simulink model "ModelVls"  (R2022b)
settings: Solver=FixedStepDiscrete  StartTime=0.0  StopTime=1  RelTol=1e-3  EnableMultiTasking=on
InitFcn:
  | % Initialize model
  | run([ModelRootName() 'Init.m']);
  | 
  | % load library data
  | GainLibrary_data;
StartFcn:
  | % make sure all the simulated RTC requests are found
  | %RTC_SIM_OBJ.ValidateREQs();
model workspace (MAT data in the model file):
  PreampVolumeTable_Idx : Simulink.Signal (value not decoded)
  Range : Simulink.Signal (value not decoded)
  Table_Idx : Simulink.Signal (value not decoded)
undefined symbols (not defined in the file): Config, Ifir, IFIR, MedusaConfig, MuteRamper, MuteRamperBtc, numAudioIn, preAmp, Row, sys_defs, VLSConfig
libraries: FeaturePath x22, TuneVar x17, RTC x9, MedusaDelays x9, dspindex x5, TOP x5, SampleRateConverter x4, EdgePorts x2, PooliirLib x2, MedusaCaeEnable x2, FIREven x2, VLSGains x2
(part 2 of 4)

== system ModelVls/PreAmp/DecRate/Medusa5H1/MedusaHoligram/Medusa5H1 Part 2 ==
  AudioIn : Inport  OutDataTypeStr=single
  LRbp : Inport  Port=2
  LRhp : Inport  Port=3
  CAEEnable : Inport  Port=4
  Alignment Delay : Subsystem  TreatAsAtomicUnit=on
      settings: RTWSystemCode=Nonreusable function  FunctionWithSeparateData=on
  Decimated-Rate FDP : MedusaFDP/Decimated-Rate  FeatureName=DeciRate  configStruct=config.DRFDPConfig  RfftConfig=[]  RifftConfig=[]
  Full-Rate FDP : MedusaFullRateFDP/Full-Rate  FeatureName=FullRate  configStruct=config.FRFDPConfig  RfftConfig=[]  RifftConfig=[]
  Mono Detector : MonoDetector/MedusaMonoDetector  Config=Config.MonoDetector
  Partition : FeaturePath/Partition  PartitionNumber=3  TriggerInit=[825 236 870 304]
      settings: SourceProductName=Bose Talaria
  SPUM Decay Estimate : MedusaSPUMDecayEst/SPUM Decay Estimate  configStruct=config.FRFDPConfig
  Selector : Selector  NumberOfDimensions=2  InputPortWidth=3  IndexOptions=Select all,Index vector (dialog)  Indices=[1 3],[1,2]  OutputSizes=1,1
  Selector1 : Selector  NumberOfDimensions=2  InputPortWidth=3  IndexOptions=Select all,Index vector (dialog)  Indices=[1 3],[1 2 3 5]  OutputSizes=1,1
  DRComps : Outport  VectorParamsAs1DForOutWhenUnconnected=off
  FRComps : Outport  Port=2  VectorParamsAs1DForOutWhenUnconnected=off
  HFRef : Outport  Port=3
  wires:
  Alignment Delay/1(LRtreble) -> Full-Rate FDP/1
  CAEEnable/1 -> Full-Rate FDP/2, Decimated-Rate FDP/2
  Selector1/1 -> HFRef/1  "Lo, Ro, Limp, Rimp"
  Full-Rate FDP/1 -> FRComps/1, Selector1/1  "Lo, Ro, Limp, Ltail, Rimp, Rtail"
  [isStereo] -> SPUM Decay Estimate/2
  LRhp/1 -> SPUM Decay Estimate/1, Alignment Delay/1(LRhp)
  LRbp/1 -> Decimated-Rate FDP/1
  AudioIn/1 -> Selector/1
  Selector/1 -> Mono Detector/1  "L, R"
  Mono Detector/1 -> [isStereo]
  SPUM Decay Estimate/1 -> Decimated-Rate FDP/3, Full-Rate FDP/3
  Decimated-Rate FDP/1 -> DRComps/1  "Lo, Ro, Ls, Rs, Limp, Ltail, Rimp, Rtail"

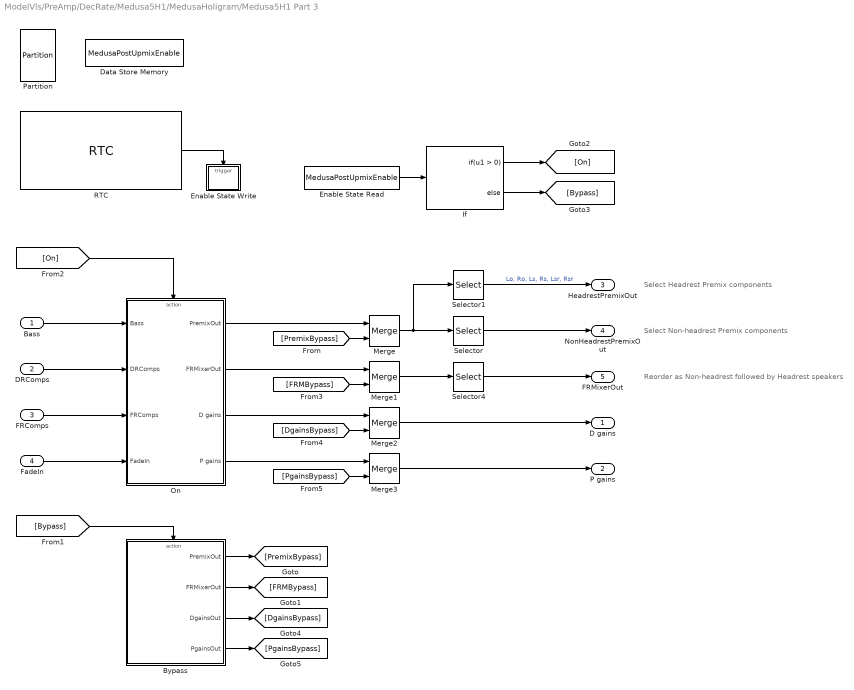
== system ModelVls/PreAmp/DecRate/Medusa5H1/MedusaHoligram/Medusa5H1 Part 3 ==
  note: Select Headrest Premix components
  note: Select Non-headrest Premix components
  note: Reorder as Non-headrest followed by Headrest speakers
  Bass : Inport
  DRComps : Inport  Port=2
  FRComps : Inport  Port=3
  FadeIn : Inport  Port=4
  Bypass : Subsystem
  Data Store Memory : DataStoreMemory  DataStoreName=MedusaPostUpmixEnable  ReadBeforeWriteMsg=warning  WriteAfterWriteMsg=warning  WriteAfterReadMsg=warning  InitialValue=1  ShowAdditionalParam=off  OutDataTypeStr=uint32
  Enable State Read : DataStoreRead  DataStoreName=MedusaPostUpmixEnable  IndexOptions=Index vector (dialog)  Indices=1  OutputSizes=1
  Enable State Write : Subsystem
  If : If
  Merge : Merge  InitialOutput=zeros(config.HoligramEQConfig.frameSize, config.PremixConfig.NumPremixOut)
  Merge1 : Merge  InitialOutput=Config.DefaultFullRateMixerOutput
  Merge2 : Merge  InitialOutput=zeros(config.numVLSGains, 1)
  Merge3 : Merge  InitialOutput=zeros(config.numVLSGains, 1)
  On : Subsystem
  Partition : FeaturePath/Partition  PartitionNumber=5  TriggerInit=[410 331 455 399]
      settings: SourceProductName=Bose Talaria
  RTC : RTC/RTC  REQ_Priority=RTC_Mask.NormalPriority  RequestAtInit=off  EnableRequest=on  REQElemType1=int32  REQElemWidth1=1  REQElemInitial1=[]  REQElemType2=uint32  REQElemWidth2=1  REQElemInitial2=[]  REQElemType3=uint32  REQElemWidth3=1  REQElemInitial3=[]  REQElemType4=uint32  REQElemWidth4=1  REQElemInitial4=[]  REQElemType5=uint32  REQElemWidth5=1  REQElemInitial5=[]  REQElemType6=uint32  REQElemWidth6=1  REQElemInitial6=[]  REQElemType7=uint32  REQElemWidth7=1  REQElemInitial7=[]  REQElemType8=uint32  REQElemWidth8=1  REQElemInitial8=[]  REQElemType9=uint32  REQElemWidth9=1  REQElemInitial9=[]  REQElemType10=uint32  REQElemWidth10=1  REQElemInitial10=[]  EnableResponse=on  EnableRSP_StatusIn=off  RSPElemType1=uint32  RSPElemWidth1=1  RSPElemType2=uint32  RSPElemWidth2=1  RSPElemType3=uint32  RSPElemWidth3=1  RSPElemType4=uint32  RSPElemWidth4=1  RSPElemType5=uint32  RSPElemWidth5=1  RSPElemType6=uint32  RSPElemWidth6=1  RSPElemType7=uint32  RSPElemWidth7=1  RSPElemType8=uint32  RSPElemWidth8=1  RSPElemType9=uint32  RSPElemWidth9=1  RSPElemType10=uint32  RSPElemWidth10=1  EnableNotification=off  EnableNTF_PrepTrig=off  NTFElemType1=uint32  NTFElemWidth1=1  NTFElemType2=uint32  NTFElemWidth2=1  NTFElemType3=uint32  NTFElemWidth3=1  NTFElemType4=uint32  NTFElemWidth4=1  NTFElemType5=uint32  NTFElemWidth5=1  NTFElemType6=uint32  NTFElemWidth6=1  NTFElemType7=uint32  NTFElemWidth7=1  NTFElemType8=uint32  NTFElemWidth8=1  NTFElemType9=uint32  NTFElemWidth9=1  NTFElemType10=uint32  NTFElemWidth10=1  MaskMessageName=PostUpmixDisable
      settings: SourceProductName=Bose Talaria
  Selector : Selector  NumberOfDimensions=2  InputPortWidth=3  IndexOptions=Select all,Index vector (dialog)  Indices=[1 3],config.NonHeadrestIdx  OutputSizes=1,1
  Selector1 : Selector  NumberOfDimensions=2  InputPortWidth=3  IndexOptions=Select all,Index vector (dialog)  Indices=[1 3],config.HeadrestIdx  OutputSizes=1,1
  Selector4 : Selector  NumberOfDimensions=2  InputPortWidth=3  IndexOptions=Select all,Index vector (dialog)  Indices=[1 3],config.FRMOutputIdx  OutputSizes=1,1
  D gains : Outport
  P gains : Outport  Port=2
  HeadrestPremixOut : Outport  Port=3  VectorParamsAs1DForOutWhenUnconnected=off
  NonHeadrestPremixOut : Outport  Port=4  VectorParamsAs1DForOutWhenUnconnected=off
  FRMixerOut : Outport  Port=5  VectorParamsAs1DForOutWhenUnconnected=off
  wires:
  Selector1/1 -> HeadrestPremixOut/1  "Lo, Ro, Ls, Rs, Lsr, Rsr"
  Selector/1 -> NonHeadrestPremixOut/1
  Merge3/1 -> P gains/1
  Merge2/1 -> D gains/1
  On/4(P gains) -> Merge3/1
  On/3(D gains) -> Merge2/1
  Merge1/1 -> Selector4/1
  On/2(FRMixerOut) -> Merge1/1
  RTC/1 -> Enable State Write/Trigger
  [On] -> On/Action
  Enable State Read/1 -> If/1
  If/2 -> [Bypass]
  If/1 -> [On]
  Merge/1 -> Selector/1, Selector1/1
  On/1(PremixOut) -> Merge/1
  [Bypass] -> Bypass/Action
  DRComps/1 -> On/2(DRComps)
  Bass/1 -> On/1(Bass)
  FRComps/1 -> On/3(FRComps)
  FadeIn/1 -> On/4(FadeIn)
  Bypass/1(PremixOut) -> [PremixBypass]
  Bypass/2(FRMixerOut) -> [FRMBypass]
  Bypass/3(DgainsOut) -> [DgainsBypass]
  Bypass/4(PgainsOut) -> [PgainsBypass]
  [PremixBypass] -> Merge/2
  [FRMBypass] -> Merge1/2
  [DgainsBypass] -> Merge2/2
  [PgainsBypass] -> Merge3/2
  Selector4/1 -> FRMixerOut/1

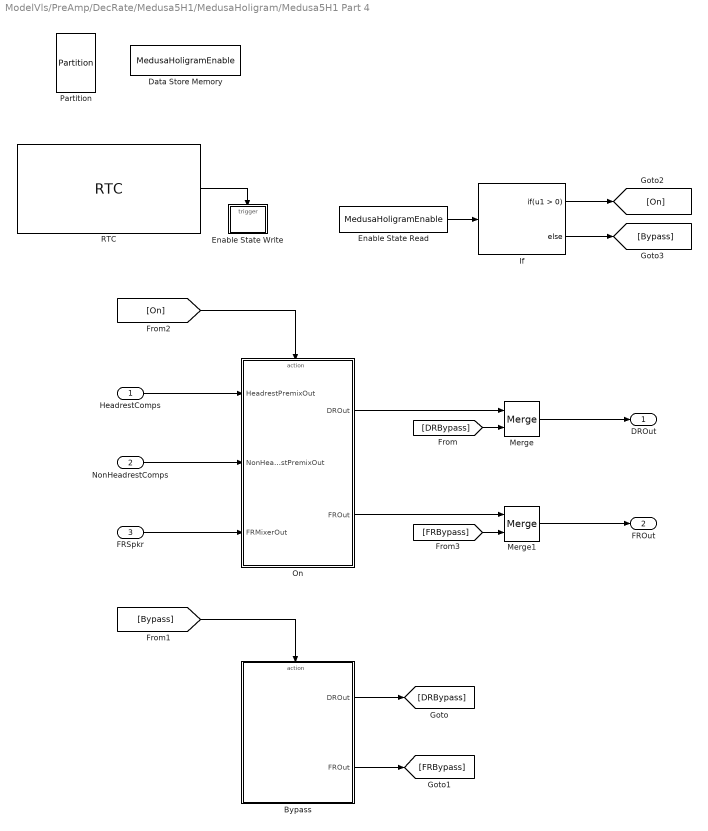
== system ModelVls/PreAmp/DecRate/Medusa5H1/MedusaHoligram/Medusa5H1 Part 4 ==
  HeadrestComps : Inport
  NonHeadrestComps : Inport  Port=2
  FRSpkr : Inport  Port=3
  Bypass : Subsystem
  Data Store Memory : DataStoreMemory  DataStoreName=MedusaHoligramEnable  ReadBeforeWriteMsg=warning  WriteAfterWriteMsg=warning  WriteAfterReadMsg=warning  InitialValue=1  ShowAdditionalParam=off  OutDataTypeStr=uint32
  Enable State Read : DataStoreRead  DataStoreName=MedusaHoligramEnable  IndexOptions=Index vector (dialog)  Indices=1  OutputSizes=1
  Enable State Write : Subsystem
  If : If
  Merge : Merge  InitialOutput=zeros(config.HoligramEQConfig.frameSize, config.numDRChan)
  Merge1 : Merge  InitialOutput=zeros(config.HoligramEQConfig.frameSizeFR, config.numMedusaOut)
  On : Subsystem
  Partition : FeaturePath/Partition  PartitionNumber=6  TriggerInit=[335 311 380 379]
      settings: SourceProductName=Bose Talaria
  RTC : RTC/RTC  REQ_Priority=RTC_Mask.NormalPriority  RequestAtInit=off  EnableRequest=on  REQElemType1=int32  REQElemWidth1=1  REQElemInitial1=[]  REQElemType2=uint32  REQElemWidth2=1  REQElemInitial2=[]  REQElemType3=uint32  REQElemWidth3=1  REQElemInitial3=[]  REQElemType4=uint32  REQElemWidth4=1  REQElemInitial4=[]  REQElemType5=uint32  REQElemWidth5=1  REQElemInitial5=[]  REQElemType6=uint32  REQElemWidth6=1  REQElemInitial6=[]  REQElemType7=uint32  REQElemWidth7=1  REQElemInitial7=[]  REQElemType8=uint32  REQElemWidth8=1  REQElemInitial8=[]  REQElemType9=uint32  REQElemWidth9=1  REQElemInitial9=[]  REQElemType10=uint32  REQElemWidth10=1  REQElemInitial10=[]  EnableResponse=on  EnableRSP_StatusIn=off  RSPElemType1=uint32  RSPElemWidth1=1  RSPElemType2=uint32  RSPElemWidth2=1  RSPElemType3=uint32  RSPElemWidth3=1  RSPElemType4=uint32  RSPElemWidth4=1  RSPElemType5=uint32  RSPElemWidth5=1  RSPElemType6=uint32  RSPElemWidth6=1  RSPElemType7=uint32  RSPElemWidth7=1  RSPElemType8=uint32  RSPElemWidth8=1  RSPElemType9=uint32  RSPElemWidth9=1  RSPElemType10=uint32  RSPElemWidth10=1  EnableNotification=off  EnableNTF_PrepTrig=off  NTFElemType1=uint32  NTFElemWidth1=1  NTFElemType2=uint32  NTFElemWidth2=1  NTFElemType3=uint32  NTFElemWidth3=1  NTFElemType4=uint32  NTFElemWidth4=1  NTFElemType5=uint32  NTFElemWidth5=1  NTFElemType6=uint32  NTFElemWidth6=1  NTFElemType7=uint32  NTFElemWidth7=1  NTFElemType8=uint32  NTFElemWidth8=1  NTFElemType9=uint32  NTFElemWidth9=1  NTFElemType10=uint32  NTFElemWidth10=1  MaskMessageName=HoligramDisable
      settings: SourceProductName=Bose Talaria
  DROut : Outport  VectorParamsAs1DForOutWhenUnconnected=off
  FROut : Outport  Port=2  VectorParamsAs1DForOutWhenUnconnected=off
  wires:
  Merge1/1 -> FROut/1
  On/2(FROut) -> Merge1/1
  RTC/1 -> Enable State Write/Trigger
  [On] -> On/Action
  Enable State Read/1 -> If/1
  If/2 -> [Bypass]
  If/1 -> [On]
  Merge/1 -> DROut/1
  On/1(DROut) -> Merge/1
  [Bypass] -> Bypass/Action
  FRSpkr/1 -> On/3(FRMixerOut)
  NonHeadrestComps/1 -> On/2(NonHeadrestPremixOut)
  HeadrestComps/1 -> On/1(HeadrestPremixOut)
  Bypass/1(DROut) -> [DRBypass]
  Bypass/2(FROut) -> [FRBypass]
  [DRBypass] -> Merge/2
  [FRBypass] -> Merge1/2

== system ModelVls/PreAmp/DecRate/Medusa5H1/MedusaHoligram/Medusa5H1 Part 5 ==
  DRIn : Inport
  FRIn : Inport  Port=2
  DR Speaker and HRComps Delay : MedusaDelays/MedusaTunableDelay  Config=Config.DeciRateSpeakerDelay
  FR Speaker Delay : MedusaDelays/MedusaTunableDelay  Config=Config.FullRateSpeakerDelay
  Partition : FeaturePath/Partition  PartitionNumber=7  TriggerInit=[1360 586 1405 654]
      settings: SourceProductName=Bose Talaria
  Speaker Delay Tune : Subsystem
  DROut : Outport  VectorParamsAs1DForOutWhenUnconnected=off
  FROut : Outport  Port=2  VectorParamsAs1DForOutWhenUnconnected=off
  wires:
  DR Speaker and HRComps Delay/1 -> DROut/1
  Speaker Delay Tune/2(FRSpeakerDelay) -> [FRSpeakerDelay]
  [DRSpeakerDelay] -> DR Speaker and HRComps Delay/2
  Speaker Delay Tune/1(DRSpeakerDelay) -> [DRSpeakerDelay]
  [FRSpeakerDelay] -> FR Speaker Delay/2
  FR Speaker Delay/1 -> FROut/1
  FRIn/1 -> FR Speaker Delay/1
  DRIn/1 -> DR Speaker and HRComps Delay/1

== system ModelVls/PreAmp/DecRate/Medusa5H1/PreAmpPart2/MuteRamperDR ==
  AudioIn : Inport
  REQ : Inport  Port=2
  NTF : Inport  Port=3
  Bus Element In2 : Inport  Port=4
  InnerLink : Subsystem  AncestorBlock=MuteRamperBtc/MuteRamper  mask(Blocklib MuteRamper){Config=InnerLinkConfig}
      mask prompts: Config "MuteRamperConfig"
      mask help: This component is to be used in conjunction with the MuteControl block, which provides runtime control and tuning capabilities via an RTC and the tune variable muteControlRampTime. Multiple instances of this block may be placed within an audio application, and a single MuteControl block has the ability to control all of these rampers simultaneously.
      mask init:
      | blkh=gcbh;
      | Config=BTConfig.Assert(blkh,Config);
      | Config.Validate();
      | 
      | % Set boundary conditions
      | rampRateBounds = [5,50000];
      | rampTimeBounds = [1,3000];
      | 
      | % Setup Dsms
      | theDsms = {'currentGain','targetLinearGain','nFrames'};
      | CscUtil.SetupDsmsForStaticInit(blkh,theDsms);
      settings: LibrarySourceBlock=MuteRamperBtc/MuteRamper
  audioOut : Outport
  NTF_check : Outport  Port=2
  wires:
  Bus Element In2/1 -> InnerLink/4(InBus)
  NTF/1 -> InnerLink/3(NTF)
  REQ/1 -> InnerLink/2(REQ)
  AudioIn/1 -> InnerLink/1(AudioIn)
  InnerLink/2(NTF_check) -> NTF_check/1
  InnerLink/1(audioOut) -> audioOut/1

== system ModelVls/PreAmp/DecRate/Medusa5H1/PreAmpPart2/MuteRamperFR ==
  AudioIn : Inport
  REQ : Inport  Port=2
  NTF : Inport  Port=3
  Bus Element In2 : Inport  Port=4
  InnerLink : Subsystem  AncestorBlock=MuteRamperBtc/MuteRamper  mask(Blocklib MuteRamper){Config=InnerLinkConfig}
      mask prompts: Config "MuteRamperConfig"
      mask help: This component is to be used in conjunction with the MuteControl block, which provides runtime control and tuning capabilities via an RTC and the tune variable muteControlRampTime. Multiple instances of this block may be placed within an audio application, and a single MuteControl block has the ability to control all of these rampers simultaneously.
      mask init: same as ModelVls/PreAmp/DecRate/Medusa5H1/PreAmpPart2/MuteRamperDR/InnerLink
      settings: LibrarySourceBlock=MuteRamperBtc/MuteRamper
  audioOut : Outport
  NTF_check : Outport  Port=2
  wires:
  Bus Element In2/1 -> InnerLink/4(InBus)
  NTF/1 -> InnerLink/3(NTF)
  REQ/1 -> InnerLink/2(REQ)
  AudioIn/1 -> InnerLink/1(AudioIn)
  InnerLink/2(NTF_check) -> NTF_check/1
  InnerLink/1(audioOut) -> audioOut/1

== system ModelVls/PreAmp/DecRate/Medusa5H1/PreAmpPart2/Subsystem ==
  In1 : Inport
  Inport : Inport  Port=2
  Trigger : TriggerPort  TriggerType=function-call  VariantControl=Variant  PortDimensions=1
  AND : Logic  IconShape=distinctive  AllPortsSameDT=off  OutDataTypeStr=boolean
  Out1 : Outport
  wires:
  In1/1 -> AND/1
  AND/1 -> Out1/1
  Inport/1 -> AND/2

== system ModelVls/PreAmp/DecRate/Medusa5H1/PreAmpPart2/Subsystem1 ==
  In1 : Inport
  Inport : Inport  Port=2
  Trigger : TriggerPort  TriggerType=function-call  VariantControl=Variant  PortDimensions=1
  AND : Logic  IconShape=distinctive  AllPortsSameDT=off  OutDataTypeStr=boolean
  Out1 : Outport
  wires:
  In1/1 -> AND/1
  AND/1 -> Out1/1
  Inport/1 -> AND/2

== system ModelVls/PreAmp/DecRate/Medusa5H1/MedusaHoligram/Medusa5H1 Part 1/CAE Treble Boost ==
  note: 1) Add Subsystem or Model blocks as valid variant choices.
      | 2) You cannot connect blocks at this level. At simulation, connectivity is automatically
      | determined, based on the active variant and port name matching.
  AudioIn : Inport
  Audio Passthrough : Subsystem  VariantControl=sys_defs.include_compressed_audio_enhancement == 0
  "CAE Treble Boost " : Subsystem  VariantControl=sys_defs.include_compressed_audio_enhancement == 1
  Out : Outport
  CAEEnable : Outport  Port=2

== system ModelVls/PreAmp/DecRate/Medusa5H1/MedusaHoligram/Medusa5H1 Part 1/Medusa Band Split Stereo ==
  LRhp : Inport
  Band Separation Delay : Delay  DelayLength=configStruct.band_separation_delay  InputProcessing=Columns as channels (frame based)
  Constant : Constant  Value=zeros(numInputs, 1)  OutDataTypeStr=uint32
  Downsample : DownSample  N=configStruct.D
  Image Rejection Filter : FIREven/FIR Even  variantSelect=Hexagon
      settings: SourceProductName=Bose Blocklib
  Image Rejection Filter Coeffs : Constant  Value=configStruct.fireven
  Interpolated Filter : Subsystem  AncestorBlock=Ifir/IFIR  mask(Interpolated FIR){coeffsFlip=configStruct.ifir, I=configStruct.D/2, numChannels=numInputs}
      mask prompts: coeffsFlip "Coefficients"; I "Interpolation Factor"; numChannels "Num inputs"
      mask help:
      | An interpolated FIR filter is an FIR filter with a sparse set of coefficients containing I-1 zeros between each point, where I is the interpolation factor.
      |
      | The block supports multiple channels, with each channel sharing the same set of filter coefficients. Users need to specify the non-zero coefficients, the interpolation factor and the number of channels.
      mask init:
      | % Flip the coeffs
      | [~, numCoeffSets] = size(coeffsFlip);
      | ind = 0:numCoeffSets-1;
      | coeffsFlip = flipud(coeffsFlip(:,ind+1));
      | 
      | % Cast decimation factor to int32
      | I = int32(I);
      settings: LibrarySourceBlock=Ifir/IFIR
  Reconstruction Filter : dspmlti4/FIR Interpolation  FilterSource=Dialog parameters  PrivateCoeffs=0  h=configStruct.upfir  L=configStruct.D  FilterObject=FINTERP  InputProcessing=Columns as channels (frame based)  framing=Enforce single-rate processing  outputBufInitCond=0  roundingMode=Floor  overflowMode=off  firstCoeffDataTypeStr=Inherit: Same word length as input  firstCoeffMin=[]  firstCoeffMax=[]  firstCoeffLastDataTypeStr=Inherit: Same word length as input  outputDataTypeStr=Inherit: Same as accumulator  outputMin=[]  outputMax=[]  outputLastDataTypeStr=Inherit: Same as accumulator
  Sum : Sum  Inputs=-+|
  LRbp : Outport  VectorParamsAs1DForOutWhenUnconnected=off
  LRtreble : Outport  Port=2  VectorParamsAs1DForOutWhenUnconnected=off
  wires:
  Constant/1 -> Image Rejection Filter/3
  Reconstruction Filter/1 -> Sum/1
  Interpolated Filter/1(AudioOut) -> Image Rejection Filter/1
  LRhp/1 -> Interpolated Filter/1(AudioIn), Band Separation Delay/1
  Image Rejection Filter Coeffs/1 -> Image Rejection Filter/2
  Image Rejection Filter/1 -> Downsample/1
  Sum/1 -> LRtreble/1
  Band Separation Delay/1 -> Sum/2
  Downsample/1 -> Reconstruction Filter/1, LRbp/1

== system ModelVls/PreAmp/DecRate/Medusa5H1/MedusaHoligram/Medusa5H1 Part 2/Alignment Delay ==
  LRhp : Inport
  Full-rate Alignment Delay Translation : MedusaDelays/MedusaFullRateAlignmentDelayTranslation  Config=Config.TrebleDelayTranslation
  Treble Delay : MedusaDelays/MedusaAlignmentDelay  Config=Config.TrebleDelay
  Tune Variable1 : TuneVar/TuneVar  TuneName=DeciRateNearWiggleFilterDelaySamples  SpecifyMaxSize=off  VariableDim=1 (Row)  MaxSize=[1 1]  TunabilityNumber=1  MinValue=[]  MaxValue=[]  TriggerInit=[-15 450 150 500]  MaskValue=Config.TrebleDelayTranslation.DefaultTuning.DeciRateNearWiggleDelay
      settings: SourceProductName=Bose Talaria
  Tune Variable4 : TuneVar/TuneVar  TuneName=DeciRateWiggleFilterDelaySamples  SpecifyMaxSize=off  VariableDim=1 (Row)  MaxSize=[1 1]  TunabilityNumber=1  MinValue=[]  MaxValue=[]  TriggerInit=[-15 385 150 435]  MaskValue=Config.TrebleDelayTranslation.DefaultTuning.DeciRateWiggleDelay
      settings: SourceProductName=Bose Talaria
  Tune Variable5 : TuneVar/TuneVar  TuneName=HoligramFilterAlignmentDelaySamples  SpecifyMaxSize=off  VariableDim=1 (Row)  MaxSize=[1 1]  TunabilityNumber=1  MinValue=[]  MaxValue=[]  TriggerInit=[-15 515 150 565]  MaskValue=Config.TrebleDelayTranslation.DefaultTuning.HoligramDelay
      settings: SourceProductName=Bose Talaria
  LRtreble : Outport
  wires:
  Tune Variable1/1 -> Full-rate Alignment Delay Translation/2  "DeciRateNearWiggleFilterDelaySamples"
  Tune Variable5/1 -> Full-rate Alignment Delay Translation/3  "HoligramFilterAlignmentDelaySamples"
  LRhp/1 -> Treble Delay/1
  Tune Variable4/1 -> Full-rate Alignment Delay Translation/1  "DeciRateWiggleFilterDelaySamples"
  Full-rate Alignment Delay Translation/1 -> [TrebleDelay]
  [TrebleDelay] -> Treble Delay/2
  Treble Delay/1 -> LRtreble/1  "LRtreble"

== system ModelVls/PreAmp/DecRate/Medusa5H1/MedusaHoligram/Medusa5H1 Part 3/Bypass ==
  Action Port : ActionPort  ActionPortLabel=else
  Constant : Constant  Value=zeros(config.HoligramEQConfig.frameSize, config.PremixConfig.NumPremixOut)  OutDataTypeStr=single
  Constant1 : Constant  Value=Config.DefaultFullRateMixerOutput  OutDataTypeStr=single
  Constant2 : Constant  Value=zeros(config.numVLSGains, 1)  OutDataTypeStr=single
  Constant3 : Constant  Value=zeros(config.numVLSGains, 1)  OutDataTypeStr=single
  PremixOut : Outport  VectorParamsAs1DForOutWhenUnconnected=off
  FRMixerOut : Outport  Port=2  VectorParamsAs1DForOutWhenUnconnected=off
  DgainsOut : Outport  Port=3  VectorParamsAs1DForOutWhenUnconnected=off
  PgainsOut : Outport  Port=4  VectorParamsAs1DForOutWhenUnconnected=off
  wires:
  Constant2/1 -> DgainsOut/1
  Constant3/1 -> PgainsOut/1
  Constant1/1 -> FRMixerOut/1
  Constant/1 -> PremixOut/1

== system ModelVls/PreAmp/DecRate/Medusa5H1/MedusaHoligram/Medusa5H1 Part 3/Enable State Write ==
  Trigger : TriggerPort  TriggerType=function-call  VariantControl=Variant  PortDimensions=1
  Constant : Constant  Value=0  OutDataTypeStr=uint32
  Data Store Write : DataStoreWrite  DataStoreName=MedusaPostUpmixEnable  IndexOptions=Index vector (dialog)  Indices=1  OutputSizes=1
  wires:
  Constant/1 -> Data Store Write/1

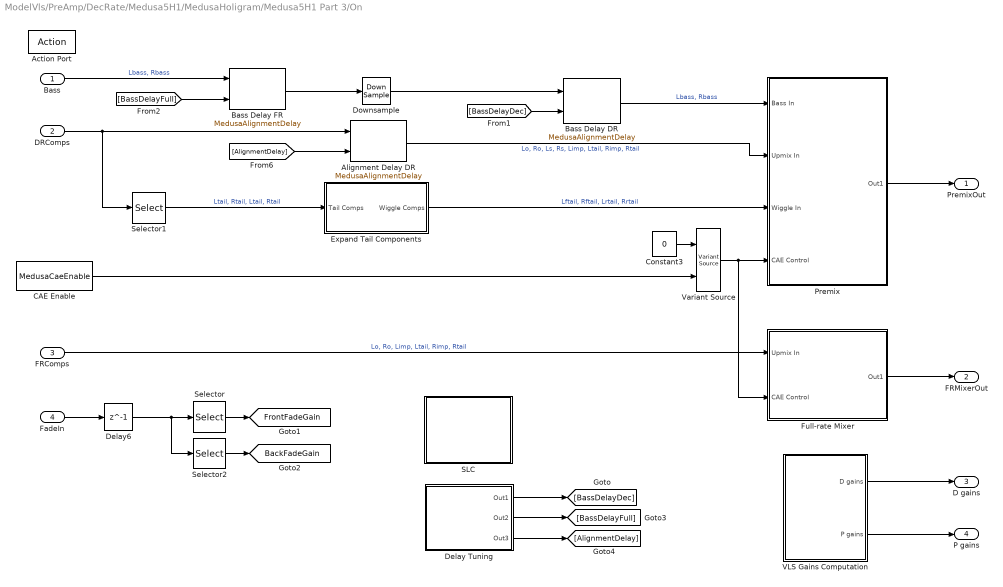
== system ModelVls/PreAmp/DecRate/Medusa5H1/MedusaHoligram/Medusa5H1 Part 3/On ==
  Bass : Inport  OutDataTypeStr=single
  DRComps : Inport  Port=2  OutDataTypeStr=single
  FRComps : Inport  Port=3  OutDataTypeStr=single
  FadeIn : Inport  Port=4  OutDataTypeStr=single
  Action Port : ActionPort  ActionPortLabel=if(u1 > 0)
  Alignment Delay DR : MedusaDelays/MedusaAlignmentDelay  Config=Config.MidrangeDelay
  Bass Delay DR : MedusaDelays/MedusaAlignmentDelay  Config=Config.DeciRateBassDelay
  Bass Delay FR : MedusaDelays/MedusaAlignmentDelay  Config=Config.FullRateBassDelay
  CAE Enable : MedusaCaeEnable/MedusaCaeEnable  Config=Config.PremixCaeEnable  MaskMessageName=PremixCAEEnable
  Constant3 : Constant  Value=0  OutDataTypeStr=int32  SampleTime=-1
  Delay Tuning : Subsystem
  Delay6 : Delay  DelayLength=1
  Downsample : DownSample  N=4
  Expand Tail Components : Subsystem  TreatAsAtomicUnit=on  RTWFileName=MedusaExpandTailComps
      settings: RTWSystemCode=Nonreusable function  RTWFileNameOpts=User specified  FunctionWithSeparateData=on
  Full-rate Mixer : Subsystem
  Premix : Subsystem
  SLC : Subsystem
  Selector : Selector  NumberOfDimensions=2  InputPortWidth=2  IndexOptions=Index vector (dialog),Index vector (dialog)  Indices=1,1  OutputSizes=1,1
  Selector1 : Selector  NumberOfDimensions=2  InputPortWidth=3  IndexOptions=Select all,Index vector (dialog)  Indices=[1 3],[6 8 6 8]  OutputSizes=1,1
  Selector2 : Selector  NumberOfDimensions=2  InputPortWidth=2  IndexOptions=Index vector (dialog),Index vector (dialog)  Indices=1,2  OutputSizes=1,1
  VLS Gains Computation : Subsystem
  Variant Source : VariantSource
  PremixOut : Outport  VectorParamsAs1DForOutWhenUnconnected=off
  FRMixerOut : Outport  Port=2  VectorParamsAs1DForOutWhenUnconnected=off
  D gains : Outport  Port=3
  P gains : Outport  Port=4
  tag scope: BackFadeGain=global, FrontFadeGain=global
  wires:
  Alignment Delay DR/1 -> Premix/2(Upmix In)  "Lo, Ro, Ls, Rs, Limp, Ltail, Rimp, Rtail"
  Variant Source/1 -> Full-rate Mixer/2(CAE Control), Premix/4(CAE Control)
  Constant3/1 -> Variant Source/1
  CAE Enable/1 -> Variant Source/2
  Full-rate Mixer/1(Out1) -> FRMixerOut/1
  FRComps/1 -> Full-rate Mixer/1(Upmix In)  "Lo, Ro, Limp, Ltail, Rimp, Rtail"
  Premix/1(Out1) -> PremixOut/1
  Expand Tail Components/1(Wiggle Comps) -> Premix/3(Wiggle In)  "Lftail, Rftail, Lrtail, Rrtail"
  Bass Delay DR/1 -> Premix/1(Bass In)  "Lbass, Rbass"
  VLS Gains Computation/2(P gains) -> P gains/1
  VLS Gains Computation/1(D gains) -> D gains/1
  Delay Tuning/3(Out3) -> [AlignmentDelay]
  Delay Tuning/2(Out2) -> [BassDelayFull]
  Delay Tuning/1(Out1) -> [BassDelayDec]
  DRComps/1 -> Alignment Delay DR/1, Selector1/1
  Downsample/1 -> Bass Delay DR/1
  [BassDelayDec] -> Bass Delay DR/2
  [AlignmentDelay] -> Alignment Delay DR/2
  [BassDelayFull] -> Bass Delay FR/2
  Bass/1 -> Bass Delay FR/1  "Lbass, Rbass"
  Selector1/1 -> Expand Tail Components/1(Tail Comps)  "Ltail, Rtail, Ltail, Rtail"
  Bass Delay FR/1 -> Downsample/1
  FadeIn/1 -> Delay6/1
  Selector2/1 -> [BackFadeGain]
  Delay6/1 -> Selector2/1, Selector/1
  Selector/1 -> [FrontFadeGain]

== system ModelVls/PreAmp/DecRate/Medusa5H1/MedusaHoligram/Medusa5H1 Part 4/Bypass ==
  Action Port : ActionPort  ActionPortLabel=else
  Constant : Constant  Value=zeros(config.HoligramEQConfig.frameSize, config.numDRChan)  OutDataTypeStr=single
  Constant1 : Constant  Value=zeros(config.HoligramEQConfig.frameSizeFR, config.numMedusaOut)  OutDataTypeStr=single
  DROut : Outport  VectorParamsAs1DForOutWhenUnconnected=off
  FROut : Outport  Port=2  VectorParamsAs1DForOutWhenUnconnected=off
  wires:
  Constant1/1 -> FROut/1
  Constant/1 -> DROut/1

== system ModelVls/PreAmp/DecRate/Medusa5H1/MedusaHoligram/Medusa5H1 Part 4/Enable State Write ==
  Trigger : TriggerPort  TriggerType=function-call  VariantControl=Variant  PortDimensions=1
  Constant : Constant  Value=0  OutDataTypeStr=uint32
  Data Store Write : DataStoreWrite  DataStoreName=MedusaHoligramEnable  IndexOptions=Index vector (dialog)  Indices=1  OutputSizes=1
  wires:
  Constant/1 -> Data Store Write/1

== system ModelVls/PreAmp/DecRate/Medusa5H1/MedusaHoligram/Medusa5H1 Part 4/On ==
  note: To fix the Headrest EQ link, FIR generic filter needs to work for multiple instances.
  HeadrestPremixOut : Inport
  NonHeadrestPremixOut : Inport  Port=2  OutDataTypeStr=single
  FRMixerOut : Inport  Port=3  OutDataTypeStr=single
  Action Port : ActionPort  ActionPortLabel=if(u1 > 0)
  DR Mix Matrix with Hybrid Holigram EQ : MedusaDRHoligramEQ/DR Holigram EQ  configStruct=config.HoligramEQConfig
  FR IIR Holigram EQ : MedusaFRHoligramEQ/FR Holigram EQ  configStruct=config.HoligramEQConfig
  Headrest Comp EQ : Subsystem  AncestorBlock=HeadrestCompEQ/Headrest Comp EQ  mask{configStruct=vlsConfigStruct.HeadrestCompEQConfig}
      mask prompts: configStruct "Config struct name:"
      mask init:
      | % Get block parameters from configStruct
      | fixedDelayLength = configStruct.fixedDelayLength;
      | IIR = configStruct.DRIIR;
      | variantFIR = configStruct.variantFIR;
      | variantIIR = configStruct.variantIIR;
      | firLength = configStruct.firLength;
      | frameSize = configStruct.frameSize;
      | numEQlink = configStruct.numEQlink;
      | numInput = configStruct.numInput;
      | 
      | % Get block default values
      | firCoeffsDefault = configStruct.firCoeffsDefault;
      | 
      | % Set implementation type for FIR
      | firBlockPath = MaskUtil.SubBlockName(gcbh, 'FIR');
      | firBlockHandle = getSimulinkBlockHandle(firBlockPath);
      | if -1 ~= firBlockHandle
      |     set_param(firBlockHandle, 'variantSelect', variantFIR);
      |     if variantFIR == 1 % Set two extras block params for Accel implementation
      |         set_param(firBlockHandle, 'numIn', num2str(numInput));
      |         set_param(firBlockHandle, 'frameSize', num2str(frameSize));
      |     end
      | end
      | 
      | iirBlockPath = MaskUtil.SubBlockName(gcbh, 'IIR');
      | iirBlockHandle = getSimulinkBlockHandle(iirBlockPath);
      | if -1 ~= iirBlockHandle
      |     set_param(iirBlockHandle, 'variantSelect', variantIIR);
      |     if variantIIR == 1 % Set two extras block params for Accel implementation
      |         set_param(iirBlockHandle, 'numChannels', num2str(numEQlink));
      |         set_param(iirBlockHandle, 'frameSize', num2str(frameSize));
      |     end
      | end
      settings: LibrarySourceBlock=HeadrestCompEQ/Headrest Comp EQ
  Matrix Concatenate : Concatenate  Mode=Multidimensional array  ConcatenateDimension=2
  DROut : Outport  VectorParamsAs1DForOutWhenUnconnected=off
  FROut : Outport  Port=2  VectorParamsAs1DForOutWhenUnconnected=off
  wires:
  FR IIR Holigram EQ/1 -> FROut/1
  Matrix Concatenate/1 -> DROut/1
  Headrest Comp EQ/1(Components Out) -> Matrix Concatenate/2
  DR Mix Matrix with Hybrid Holigram EQ/1 -> Matrix Concatenate/1
  FRMixerOut/1 -> FR IIR Holigram EQ/1
  NonHeadrestPremixOut/1 -> DR Mix Matrix with Hybrid Holigram EQ/1
  HeadrestPremixOut/1 -> Headrest Comp EQ/1(Components In)

== system ModelVls/PreAmp/DecRate/Medusa5H1/MedusaHoligram/Medusa5H1 Part 5/Speaker Delay Tune ==
  Output Delay Translation with Headrest : MedusaDelays/HeadrestOutputDelayTranslation  Config=[]
  TOP3 : TOP/TOP  TriggerInit=[645 305 895 365]  TopName=FRSpeakerDelay  DataType=int32  BankNumber=0  PreOverlay=false  PostOverlay=false  Role=Automatic
      settings: SourceProductName=Bose Talaria
  TOP5 : TOP/TOP  TriggerInit=[645 155 895 215]  TopName=DRSpeakerDelay  DataType=int32  BankNumber=0  PreOverlay=false  PostOverlay=false  Role=Automatic
      settings: SourceProductName=Bose Talaria
  Tune Variable : TuneVar/TuneVar  TuneName=HeadrestDrvSpeakerDelaySamples  SpecifyMaxSize=off  VariableDim=1 (Row)  MaxSize=[1 1]  TunabilityNumber=1  MinValue=[]  MaxValue=[]  TriggerInit=[20 195 245 245]  MaskValue=[0]
      settings: SourceProductName=Bose Talaria
  Tune Variable1 : TuneVar/TuneVar  TuneName=NonHeadrestSpeakerDelaySamples  SpecifyMaxSize=off  VariableDim=1 (Row)  MaxSize=[1 1]  TunabilityNumber=1  MinValue=[]  MaxValue=[]  TriggerInit=[20 120 245 170]  MaskValue=HRDelayConfig.DRNonHRDelay
      settings: SourceProductName=Bose Talaria
  Tune Variable4 : TuneVar/TuneVar  TuneName=HeadrestPaxSpeakerDelaySamples  SpecifyMaxSize=off  VariableDim=1 (Row)  MaxSize=[1 1]  TunabilityNumber=1  MinValue=[]  MaxValue=[]  TriggerInit=[20 270 245 320]  MaskValue=[0]
      settings: SourceProductName=Bose Talaria
  Tune Variable5 : TuneVar/TuneVar  TuneName=FRHoligramDelaySamples  SpecifyMaxSize=off  VariableDim=1 (Row)  MaxSize=[]  TunabilityNumber=1  MinValue=[]  MaxValue=[]  TriggerInit=[20 345 245 395]  MaskValue=HRDelayConfig.FRSpkrDelay
      settings: SourceProductName=Bose Talaria
  DRSpeakerDelay : Outport
  FRSpeakerDelay : Outport  Port=2
  wires:
  Output Delay Translation with Headrest/2 -> TOP3/1
  Output Delay Translation with Headrest/1 -> TOP5/1
  Tune Variable5/1 -> Output Delay Translation with Headrest/4  "FRHoligramDelaySamples"
  Tune Variable4/1 -> Output Delay Translation with Headrest/3  "HeadrestPaxSpeakerDelaySamples"
  Tune Variable/1 -> Output Delay Translation with Headrest/2  "HeadrestDrvSpeakerDelaySamples"
  Tune Variable1/1 -> Output Delay Translation with Headrest/1  "NonHeadrestSpeakerDelaySamples"
  TOP3/1 -> FRSpeakerDelay/1  "FRSpeakerDelay"
  TOP5/1 -> DRSpeakerDelay/1  "DRSpeakerDelay"

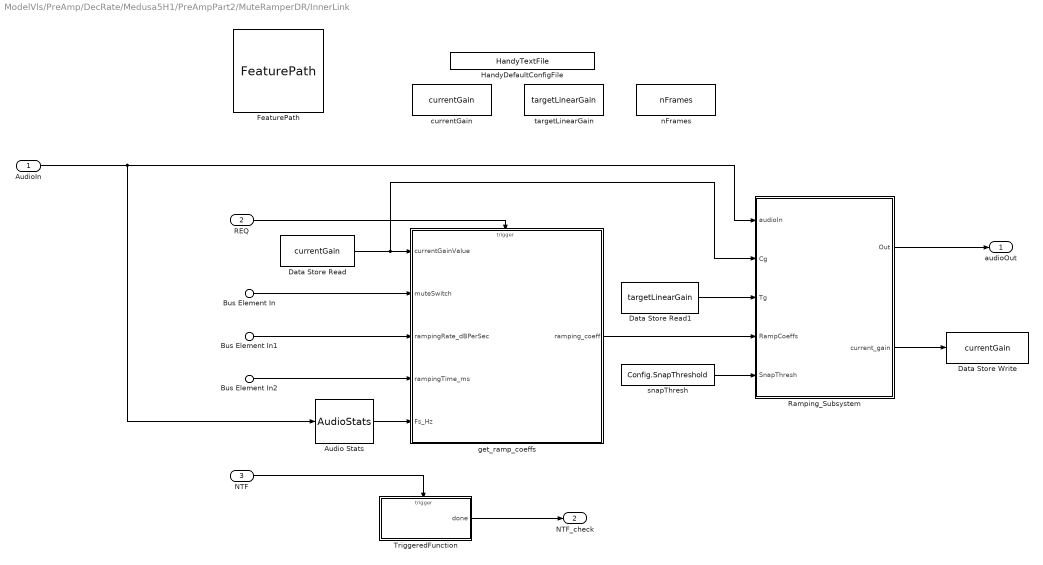
== system ModelVls/PreAmp/DecRate/Medusa5H1/PreAmpPart2/MuteRamperDR/InnerLink ==
  AudioIn : Inport
  REQ : Inport  Port=2
  NTF : Inport  Port=3
  Bus Element In : Inport  Port=4  PortName=InBus  Element=REQ_mute_switch
  Bus Element In1 : Inport  Port=4  PortName=InBus  Element=rampRate
  Bus Element In2 : Inport  Port=4  PortName=InBus  Element=rampTime
  Audio Stats : AudioStats/AudioStats  DoSampleRate=on  TypeSampleRate=Inherit: auto  DoCallRate=off  TypeCallRate=Inherit: auto  DoFrameSize=off  TypeFrameSize=Inherit: auto  DoChannelCount=off  TypeChannelCount=Inherit: auto  DoTaskRateFactor=off  TypeTaskRateFactor=Inherit: auto  MacroNameRoot=AUDIO  MacroNameRootEval='AUDIO'  IsMacroNameEval=off  MacroSampleRate=off  MacroCallRate=off  MacroFrameSize=off  MacroChannelCount=off  MacroTaskRateFactor=off  MacroTaskId=off  ValidateSampleRate=off  ValueSampleRate=[]  ValidateCallRate=off  ValueCallRate=[]  ValidateFrameSize=off  ValueFrameSize=[]  ValidateChannelCount=off  ValueChannelCount=[]  ValidateTaskRateFactor=off  ValueTaskRateFactor=[]
      settings: SourceProductName=Bose Talaria
  Data Store Read : DataStoreRead  DataStoreName=currentGain  IndexOptions=Index vector (dialog)  Indices=1  OutputSizes=1
  Data Store Read1 : DataStoreRead  DataStoreName=targetLinearGain  IndexOptions=Index vector (dialog)  Indices=1  OutputSizes=1
  Data Store Write : DataStoreWrite  DataStoreName=currentGain  IndexOptions=Index vector (dialog)  Indices=1  OutputSizes=1
  FeaturePath : FeaturePath/FeaturePath  FeatureName=MuteRamperDR  IsGroup=off  GroupNumber=-1  IsModule=off  TriggerInit=[730 -51 845 56]
      settings: SourceProductName=Bose Talaria
  HandyDefaultConfigFile : HandyTextFile/HandyTextFile  TemplateSource=Config  FileSuffix=Init  OpenDialogOnLoad=off  UseThisBlockName=off  AddGrandParentNamePrefix=off  TheDefaultText=|  ShowInLibBrowser=on
      | % $(FILENAME) Setup model parameters for each "Init" callback (e.g. update diagram)
      | sample_rate_in_hertz = 44100;
      | frame_size = 32;
      | sysin_channel_count = 2;
      settings: SourceProductName=Bose Talaria
  Ramping_Subsystem : Subsystem  TreatAsAtomicUnit=on
  TriggeredFunction : MATLAB Function  TreatAsAtomicUnit=on
  currentGain : DataStoreMemory  DataStoreName=currentGain  InitialValue=Config.DlgInitialGainLinear  ShowAdditionalParam=off  OutDataTypeStr=single
  get_ramp_coeffs : MATLAB Function  TreatAsAtomicUnit=on  mask{silentGainLinear=Config.SilentGainLinear, frameSize=Config.SamplesPerFrame}
  nFrames : DataStoreMemory  DataStoreName=nFrames  ShowAdditionalParam=off  OutDataTypeStr=single
  snapThresh : Constant  Value=Config.SnapThreshold  VectorParams1D=off  OutDataTypeStr=single
  targetLinearGain : DataStoreMemory  DataStoreName=targetLinearGain  InitialValue=Config.DlgInitialGainLinear  ShowAdditionalParam=off  OutDataTypeStr=single
  audioOut : Outport  VectorParamsAs1DForOutWhenUnconnected=off
  NTF_check : Outport  Port=2
  wires:
  Data Store Read/1 -> get_ramp_coeffs/1(currentGainValue), Ramping_Subsystem/2(Cg)
  Bus Element In1/1 -> get_ramp_coeffs/3(rampingRate_dBPerSec)
  AudioIn/1 -> Ramping_Subsystem/1(audioIn), Audio Stats/1
  Ramping_Subsystem/1(Out) -> audioOut/1
  get_ramp_coeffs/1(ramping_coeff) -> Ramping_Subsystem/4(RampCoeffs)
  Data Store Read1/1 -> Ramping_Subsystem/3(Tg)
  Bus Element In2/1 -> get_ramp_coeffs/4(rampingTime_ms)
  Ramping_Subsystem/2(current_gain) -> Data Store Write/1
  Bus Element In/1 -> get_ramp_coeffs/2(muteSwitch)
  TriggeredFunction/1(done) -> NTF_check/1
  NTF/1 -> TriggeredFunction/Trigger
  Audio Stats/1 -> get_ramp_coeffs/5(Fs_Hz)
  snapThresh/1 -> Ramping_Subsystem/5(SnapThresh)
  REQ/1 -> get_ramp_coeffs/Trigger

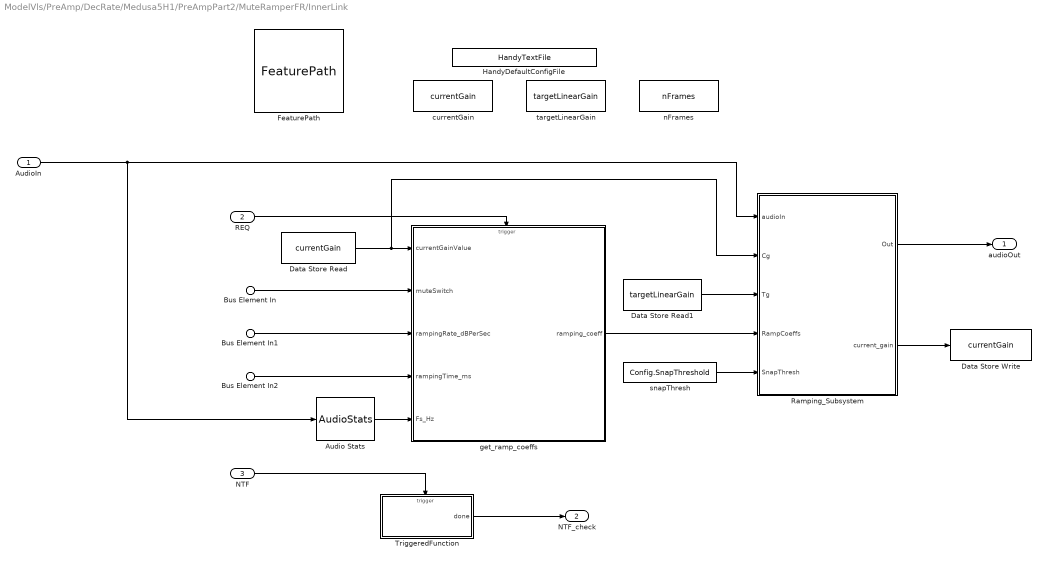
== system ModelVls/PreAmp/DecRate/Medusa5H1/PreAmpPart2/MuteRamperFR/InnerLink ==
  AudioIn : Inport
  REQ : Inport  Port=2
  NTF : Inport  Port=3
  Bus Element In : Inport  Port=4  PortName=InBus  Element=REQ_mute_switch
  Bus Element In1 : Inport  Port=4  PortName=InBus  Element=rampRate
  Bus Element In2 : Inport  Port=4  PortName=InBus  Element=rampTime
  Audio Stats : AudioStats/AudioStats  DoSampleRate=on  TypeSampleRate=Inherit: auto  DoCallRate=off  TypeCallRate=Inherit: auto  DoFrameSize=off  TypeFrameSize=Inherit: auto  DoChannelCount=off  TypeChannelCount=Inherit: auto  DoTaskRateFactor=off  TypeTaskRateFactor=Inherit: auto  MacroNameRoot=AUDIO  MacroNameRootEval='AUDIO'  IsMacroNameEval=off  MacroSampleRate=off  MacroCallRate=off  MacroFrameSize=off  MacroChannelCount=off  MacroTaskRateFactor=off  MacroTaskId=off  ValidateSampleRate=off  ValueSampleRate=[]  ValidateCallRate=off  ValueCallRate=[]  ValidateFrameSize=off  ValueFrameSize=[]  ValidateChannelCount=off  ValueChannelCount=[]  ValidateTaskRateFactor=off  ValueTaskRateFactor=[]
      settings: SourceProductName=Bose Talaria
  Data Store Read : DataStoreRead  DataStoreName=currentGain  IndexOptions=Index vector (dialog)  Indices=1  OutputSizes=1
  Data Store Read1 : DataStoreRead  DataStoreName=targetLinearGain  IndexOptions=Index vector (dialog)  Indices=1  OutputSizes=1
  Data Store Write : DataStoreWrite  DataStoreName=currentGain  IndexOptions=Index vector (dialog)  Indices=1  OutputSizes=1
  FeaturePath : FeaturePath/FeaturePath  FeatureName=MuteRamperFR  IsGroup=off  GroupNumber=-1  IsModule=off  TriggerInit=[755 -46 870 61]
      settings: SourceProductName=Bose Talaria
  HandyDefaultConfigFile : HandyTextFile/HandyTextFile  TemplateSource=Config  FileSuffix=Init  OpenDialogOnLoad=off  UseThisBlockName=off  AddGrandParentNamePrefix=off  TheDefaultText=|  ShowInLibBrowser=on
      | % $(FILENAME) Setup model parameters for each "Init" callback (e.g. update diagram)
      | sample_rate_in_hertz = 44100;
      | frame_size = 32;
      | sysin_channel_count = 2;
      settings: SourceProductName=Bose Talaria
  Ramping_Subsystem : Subsystem  TreatAsAtomicUnit=on
  TriggeredFunction : MATLAB Function  TreatAsAtomicUnit=on
  currentGain : DataStoreMemory  DataStoreName=currentGain  InitialValue=Config.DlgInitialGainLinear  ShowAdditionalParam=off  OutDataTypeStr=single
  get_ramp_coeffs : MATLAB Function  TreatAsAtomicUnit=on  mask{silentGainLinear=Config.SilentGainLinear, frameSize=Config.SamplesPerFrame}
  nFrames : DataStoreMemory  DataStoreName=nFrames  ShowAdditionalParam=off  OutDataTypeStr=single
  snapThresh : Constant  Value=Config.SnapThreshold  VectorParams1D=off  OutDataTypeStr=single
  targetLinearGain : DataStoreMemory  DataStoreName=targetLinearGain  InitialValue=Config.DlgInitialGainLinear  ShowAdditionalParam=off  OutDataTypeStr=single
  audioOut : Outport  VectorParamsAs1DForOutWhenUnconnected=off
  NTF_check : Outport  Port=2
  wires:
  Data Store Read/1 -> get_ramp_coeffs/1(currentGainValue), Ramping_Subsystem/2(Cg)
  Bus Element In1/1 -> get_ramp_coeffs/3(rampingRate_dBPerSec)
  AudioIn/1 -> Ramping_Subsystem/1(audioIn), Audio Stats/1
  Ramping_Subsystem/1(Out) -> audioOut/1
  get_ramp_coeffs/1(ramping_coeff) -> Ramping_Subsystem/4(RampCoeffs)
  Data Store Read1/1 -> Ramping_Subsystem/3(Tg)
  Bus Element In2/1 -> get_ramp_coeffs/4(rampingTime_ms)
  Ramping_Subsystem/2(current_gain) -> Data Store Write/1
  Bus Element In/1 -> get_ramp_coeffs/2(muteSwitch)
  TriggeredFunction/1(done) -> NTF_check/1
  NTF/1 -> TriggeredFunction/Trigger
  Audio Stats/1 -> get_ramp_coeffs/5(Fs_Hz)
  snapThresh/1 -> Ramping_Subsystem/5(SnapThresh)
  REQ/1 -> get_ramp_coeffs/Trigger

== system ModelVls/PreAmp/DecRate/Medusa5H1/MedusaHoligram/Medusa5H1 Part 1/CAE Treble Boost/Audio Passthrough ==
  AudioIn : Inport
  Constant : Constant  Value=0  OutDataTypeStr=int32  SampleTime=-1
  Constant3 : Constant  Value=0  OutDataTypeStr=int32  SampleTime=-1
  Target StateVar : StateVar/TargetStateVar  TriggerInit=[235 166 375 234]  TspName=DummyState  StateName=DummyState  UseSameName=on  IfdefMacro=[]
      settings: SourceProductName=Bose Talaria
  Terminator : Terminator
  TuneTOP : TuneVar/TuneTOP  TriggerInit=[50 262 220 318]  TopName=DummyTune  TuneName=DummyTune  DataType=single  TunabilityNumber=1  MinValue=[]  MaxValue=[]  BankNumber=0  PreOverlay=false  PostOverlay=false  UseSameName=on  MaskValue=[1]
      settings: SourceProductName=Bose Talaria
  Out : Outport
  CAEEnable : Outport  Port=2
  wires:
  Constant3/1 -> CAEEnable/1
  Constant/1 -> Target StateVar/1
  TuneTOP/1 -> Terminator/1
  AudioIn/1 -> Out/1

== system ModelVls/PreAmp/DecRate/Medusa5H1/MedusaHoligram/Medusa5H1 Part 1/CAE Treble Boost/CAE Treble Boost  ==
  AudioIn : Inport
  CAE Enable : MedusaCaeEnable/MedusaCaeEnable  Config=Config.CaeEnable  MaskMessageName=CAEEnable
  Treble Boost : TrebleBoost/TrebleBoostStereo  Config=Config.TrebleBoost
  Tune Variable4 : TuneVar/TuneVar  Description=|  TuneName=SurroundOn  SpecifyMaxSize=off  VariableDim=1 (Row)  MaxSize=[1 1]  TunabilityNumber=1  MinValue=[]  MaxValue=[]  TriggerInit=[-50 35 120 85]  MaskValue=2
      | General surround control parameter
      | STEREO_MODE = 0
      | SURROUND_PASSTHRU_MODE = 1
      | MEDUSA_2_CHANNEL_MODE = 2
      | MEDUSA_5_1_MODE = 3
      settings: SourceProductName=Bose Talaria
  Out : Outport
  CAEEnable : Outport  Port=2
  wires:
  Treble Boost/1 -> Out/1
  AudioIn/1 -> Treble Boost/1
  Tune Variable4/1 -> Treble Boost/2  "SurroundOn"
  CAE Enable/1 -> CAEEnable/1, Treble Boost/3

== system ModelVls/PreAmp/DecRate/Medusa5H1/MedusaHoligram/Medusa5H1 Part 1/Medusa Band Split Stereo/Interpolated Filter ==
  AudioIn : Inport
  Data Store Memory : DataStoreMemory  DataStoreName=states  ReadBeforeWriteMsg=warning  WriteAfterWriteMsg=warning  WriteAfterReadMsg=warning  InitialValue=zeros(size(coeffsFlip,1)*I,numChannels)  ShowAdditionalParam=off  OutDataTypeStr=single
  ifir : MATLAB Function  TreatAsAtomicUnit=on
  AudioOut : Outport  VectorParamsAs1DForOutWhenUnconnected=off
  wires:
  ifir/1(audioOut) -> AudioOut/1
  AudioIn/1 -> ifir/1(audioIn)

== system ModelVls/PreAmp/DecRate/Medusa5H1/MedusaHoligram/Medusa5H1 Part 3/On/Delay Tuning ==
  Delay Translation : MedusaDelays/MedusaAlignmentDelayTranslation  Config=Config.AlignmentDelayTranslation
  Tune Variable : TuneVar/TuneVar  TuneName=WiggleFilterDelayDecRateSamples1  SpecifyMaxSize=off  VariableDim=1 (Row)  MaxSize=[1 1]  TunabilityNumber=1  MinValue=[]  MaxValue=[]  TriggerInit=[-115 25 55 75]  MaskValue=Config.AlignmentDelayTranslation.DefaultTuning.DeciRateWiggleDelay
      settings: SourceProductName=Bose Talaria
  Tune Variable1 : TuneVar/TuneVar  TuneName=NEARWiggleFilterDelayDecRateSamples1  SpecifyMaxSize=off  VariableDim=1 (Row)  MaxSize=[1 1]  TunabilityNumber=1  MinValue=[]  MaxValue=[]  TriggerInit=[-115 87 55 133]  MaskValue=Config.AlignmentDelayTranslation.DefaultTuning.DeciRateNearWiggleDelay
      settings: SourceProductName=Bose Talaria
  Out1 : Outport
  Out2 : Outport  Port=2
  Out3 : Outport  Port=3
  wires:
  Tune Variable1/1 -> Delay Translation/2  "NEARWiggleFilterDelayDecRateSamples1"
  Delay Translation/3 -> Out3/1
  Delay Translation/1 -> Out1/1
  Delay Translation/2 -> Out2/1
  Tune Variable/1 -> Delay Translation/1  "WiggleFilterDelayDecRateSamples1"

== system ModelVls/PreAmp/DecRate/Medusa5H1/MedusaHoligram/Medusa5H1 Part 3/On/Expand Tail Components ==
  Tail Comps : Inport
  Constant : Constant  Value=[0 1 2 3]  OutDataTypeStr=single  SampleTime=-1
  Tail Component EQ : PooliirLib/PooliirwithNonTrivialTranslations  maxNumStages=tailCompEQ.maxNumStages  numStages=tailCompEQ.numStages  sosCoefficients=tailCompEQ.coeffs  FeatureName=tailCompEQ
  TuneTOP : TuneVar/TuneTOP  TriggerInit=[265 167 435 223]  TopName=WiggleFilter  TuneName=WiggleFilter  DataType=single  TunabilityNumber=1  MinValue=[]  MaxValue=[]  BankNumber=0  PreOverlay=false  PostOverlay=false  UseSameName=on  MaskValue=config.wiggleFilterDefault
      settings: SourceProductName=Bose Talaria
  Wiggle Filters : FIREven/FIR Even  variantSelect=Hexagon
      settings: SourceProductName=Bose Blocklib
  Wiggle Comps : Outport  VectorParamsAs1DForOutWhenUnconnected=off
  wires:
  Tail Comps/1 -> Wiggle Filters/1  "Ltail, Rtail, Ltail, Rtail"
  Tail Component EQ/1 -> Wiggle Comps/1
  Constant/1 -> Wiggle Filters/3
  TuneTOP/1 -> [wiggleFilter]
  Wiggle Filters/1 -> Tail Component EQ/1  "Lftail, Rftail, Lrtail, Rrtail"
  [wiggleFilter] -> Wiggle Filters/2

== system ModelVls/PreAmp/DecRate/Medusa5H1/MedusaHoligram/Medusa5H1 Part 3/On/Full-rate Mixer ==
  Upmix In : Inport
  CAE Control : Inport  Port=2
  Full-Rate Mixer with CAE & Fade Ramper : MedusaFullRateMixer/Full-Rate Mixer with CAE & Fade Ramper  MedusaFRMConfig=config.FRMConfig  MedusaFRMTune=config.FRMTune
  Out1 : Outport
  tag scope: NTFDone2=global
  wires:
  CAE Control/1 -> Full-Rate Mixer with CAE & Fade Ramper/9
  [SLC_On] -> Full-Rate Mixer with CAE & Fade Ramper/5
  [NTFCheck2] -> Full-Rate Mixer with CAE & Fade Ramper/8
  [BackFadeGain] -> Full-Rate Mixer with CAE & Fade Ramper/3
  [SurroundInfo] -> Full-Rate Mixer with CAE & Fade Ramper/7
  [SLCTrigger2] -> Full-Rate Mixer with CAE & Fade Ramper/6
  Full-Rate Mixer with CAE & Fade Ramper/2 -> [NTFDone2]
  [SLCReset2] -> Full-Rate Mixer with CAE & Fade Ramper/4
  [FrontFadeGain] -> Full-Rate Mixer with CAE & Fade Ramper/2
  Full-Rate Mixer with CAE & Fade Ramper/1 -> Out1/1
  Upmix In/1 -> Full-Rate Mixer with CAE & Fade Ramper/1

== system ModelVls/PreAmp/DecRate/Medusa5H1/MedusaHoligram/Medusa5H1 Part 3/On/Premix ==
  Bass In : Inport
  Upmix In : Inport  Port=2
  Wiggle In : Inport  Port=3
  CAE Control : Inport  Port=4
  Premix with Mono-Surround & CAE with Fade Ramper : MedusaPremix/PremixWithMonoSurroundAndCaeWithFadeRamper  MedusaPremixConfig=config.PremixConfig  MedusaPremixTune=config.PremixTune  MSConfig=config.MSConfig
  Out1 : Outport
  tag scope: NTFDone1=global
  wires:
  [SLC_On] -> Premix with Mono-Surround & CAE with Fade Ramper/7
  CAE Control/1 -> Premix with Mono-Surround & CAE with Fade Ramper/11
  Premix with Mono-Surround & CAE with Fade Ramper/1 -> Out1/1
  Premix with Mono-Surround & CAE with Fade Ramper/2 -> [NTFDone1]
  Upmix In/1 -> Premix with Mono-Surround & CAE with Fade Ramper/2
  Wiggle In/1 -> Premix with Mono-Surround & CAE with Fade Ramper/3
  [BackFadeGain] -> Premix with Mono-Surround & CAE with Fade Ramper/5
  [NTFCheck1] -> Premix with Mono-Surround & CAE with Fade Ramper/10
  [SLCReset1] -> Premix with Mono-Surround & CAE with Fade Ramper/6
  [SLCTrigger1] -> Premix with Mono-Surround & CAE with Fade Ramper/8
  [FrontFadeGain] -> Premix with Mono-Surround & CAE with Fade Ramper/4
  [SurroundInfo] -> Premix with Mono-Surround & CAE with Fade Ramper/9
  Bass In/1 -> Premix with Mono-Surround & CAE with Fade Ramper/1

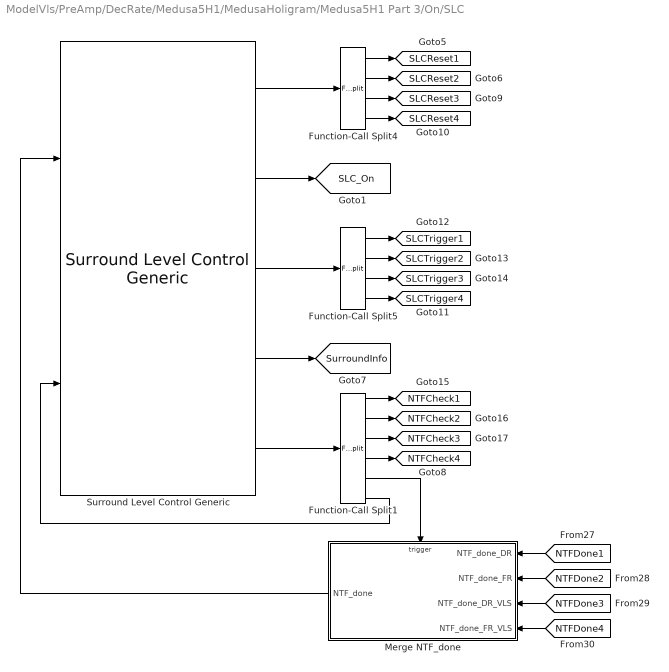
== system ModelVls/PreAmp/DecRate/Medusa5H1/MedusaHoligram/Medusa5H1 Part 3/On/SLC ==
  Function-Call Split1 : FunctionCallSplit  IconShape=distinctive  NumOutputPorts=6  OutputPortLayout=default
  Function-Call Split4 : FunctionCallSplit  IconShape=distinctive  NumOutputPorts=4  OutputPortLayout=default
  Function-Call Split5 : FunctionCallSplit  IconShape=distinctive  NumOutputPorts=4  OutputPortLayout=default
  Merge NTF_done : Subsystem
  Surround Level Control Generic : MedusaSurroundLevelControl/Surround Level Control Generic  SurroundConfig=config.SurroundConfig
  tag scope: NTFCheck1=global, NTFCheck2=global, NTFCheck3=global, NTFCheck4=global, SLCReset1=global, SLCReset2=global, SLCReset3=global, SLCReset4=global, SLCTrigger1=global, SLCTrigger2=global, SLCTrigger3=global, SLCTrigger4=global, SLC_On=global, SurroundInfo=global
  wires:
  Function-Call Split1/6 -> Surround Level Control Generic/2
  Surround Level Control Generic/2 -> [SLC_On]
  Surround Level Control Generic/5 -> Function-Call Split1/1
  Merge NTF_done/1(NTF_done) -> Surround Level Control Generic/1
  [NTFDone3] -> Merge NTF_done/3(NTF_done_DR_VLS)
  Function-Call Split4/4 -> [SLCReset4]
  Function-Call Split5/3 -> [SLCTrigger3]
  Function-Call Split5/1 -> [SLCTrigger1]
  Surround Level Control Generic/3 -> Function-Call Split5/1
  Surround Level Control Generic/4 -> [SurroundInfo]
  Function-Call Split4/1 -> [SLCReset1]
  Function-Call Split5/4 -> [SLCTrigger4]
  Function-Call Split4/3 -> [SLCReset3]
  [NTFDone4] -> Merge NTF_done/4(NTF_done_FR_VLS)
  Function-Call Split1/5 -> Merge NTF_done/Trigger
  Function-Call Split4/2 -> [SLCReset2]
  [NTFDone2] -> Merge NTF_done/2(NTF_done_FR)
  Function-Call Split1/4 -> [NTFCheck4]
  Function-Call Split5/2 -> [SLCTrigger2]
  Function-Call Split1/2 -> [NTFCheck2]
  Function-Call Split1/1 -> [NTFCheck1]
  [NTFDone1] -> Merge NTF_done/1(NTF_done_DR)
  Surround Level Control Generic/1 -> Function-Call Split4/1
  Function-Call Split1/3 -> [NTFCheck3]

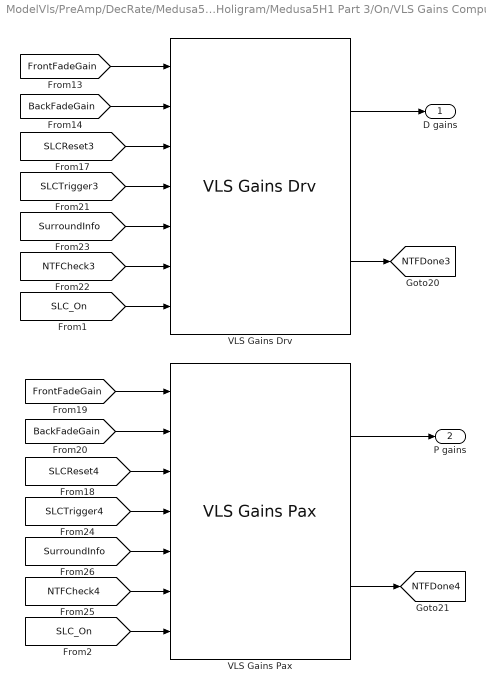
== system ModelVls/PreAmp/DecRate/Medusa5H1/MedusaHoligram/Medusa5H1 Part 3/On/VLS Gains Computation ==
  VLS Gains Drv : VLSGains/VLS Gains Drv  configStruct=vlsConfigStruct.VLSGainsConfig  tuneStruct=vlsConfigStruct.VLSGainsTune  FeatureName=VLSDrvGains
  VLS Gains Pax : VLSGains/VLS Gains Pax  configStruct=vlsConfigStruct.VLSGainsConfig  tuneStruct=vlsConfigStruct.VLSGainsTune  FeatureName=VLSPaxGains
  D gains : Outport
  P gains : Outport  Port=2
  tag scope: NTFDone3=global, NTFDone4=global
  wires:
  [SLC_On] -> VLS Gains Pax/7
  [SLC_On] -> VLS Gains Drv/7
  VLS Gains Pax/1 -> P gains/1
  VLS Gains Drv/1 -> D gains/1
  [FrontFadeGain] -> VLS Gains Drv/1
  [SLCReset4] -> VLS Gains Pax/3
  [SLCTrigger4] -> VLS Gains Pax/4
  [FrontFadeGain] -> VLS Gains Pax/1
  [SurroundInfo] -> VLS Gains Pax/5
  [NTFCheck4] -> VLS Gains Pax/6
  [BackFadeGain] -> VLS Gains Drv/2
  [SLCTrigger3] -> VLS Gains Drv/4
  VLS Gains Drv/2 -> [NTFDone3]
  VLS Gains Pax/2 -> [NTFDone4]
  [SurroundInfo] -> VLS Gains Drv/5
  [BackFadeGain] -> VLS Gains Pax/2
  [SLCReset3] -> VLS Gains Drv/3
  [NTFCheck3] -> VLS Gains Drv/6
